simulink model "sampleModel228"  (R2021b)
settings: Solver=VariableStepAuto  StartTime=0.0  StopTime=10.0  RelTol=1e-3
undefined symbols (not defined in the file or in its folder): DiscIntNeverNeededParam
settings Model: Creator=user  LastModifiedBy=user

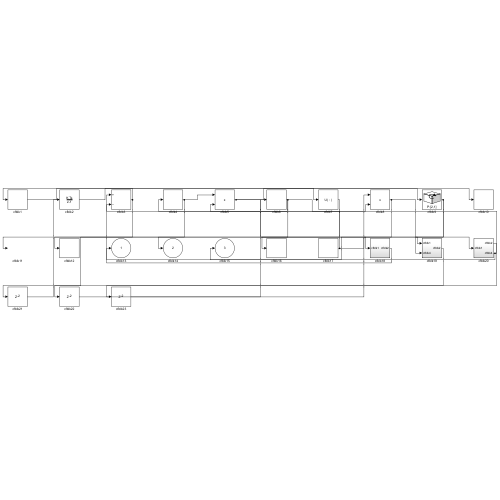
[thumbnail: Simulink's stored preview of the top-level diagram]
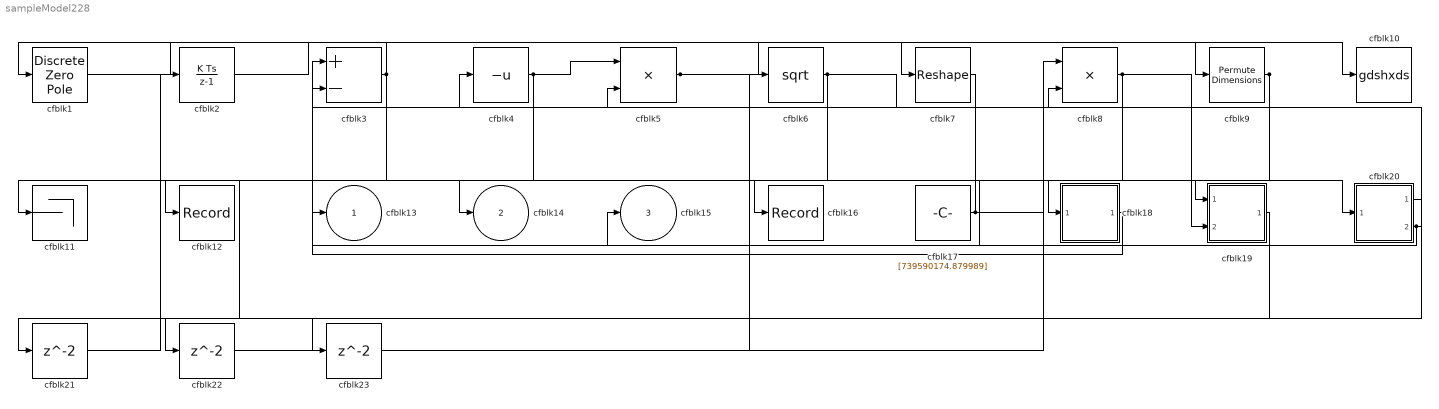
== system sampleModel228 ==
  cfblk1 : DiscreteZeroPole  Poles=[0 0.5]  Gain=1
  cfblk10 : ToWorkspace  VariableName=gdshxds  SaveFormat=Timeseries  SampleTime=-1
  cfblk11 : Terminator
  cfblk12 : Record  FileSettingsInternal="{\"entries\":[{\"content\":{\"excelSettings\":{\"content\":{},\"type\":\"Streamout.ExcelSettings\"}},\"type\":\"Streamout.FileSettingStorage\",\"uuid\":\"b7853067-aa81-4ff4-b03c-5eefb2e9456f\"}],\"packageUris\":[\"http://schema.mathworks.com/mf0/streamout_blocks/R2020a\"],\"version\":\"1.0\"}"  SignalsInternal="{\"entries\":[{\"content\":{\"signals\":[{\"content\":{\"blockPath\":[\"sampleModel228/cfblk12\"],\"channel\":[],\"dimensions\":[1,1],\"domain\":\"sampleModel228/cfblk12\",\"lineColor\":\"#edb120\",\"plots\":[1],\"port\":1,\"sid\":[\"\"],\"signalID\":8909,\"signalName\":\"cfblk3\"},\"type\":\"RecordBlkView.Signal\",\"uuid\":\"a36b1164-e6c3-447c-bebc-b7c5e35fa2b4\"}]},\"type\":\"RecordBlkView.InputSignals\",\"uuid\":\"7dc5b746-0d92-4986-ba98-2d25609e5927\"}],\"packageUris\":[\"http://schema.mathworks.com/mf0/streamout_blocks/R2020a\"],\"version\":\"1.0\"}"  VisualizationBindings="{\"sparklinesplugin\":{\"info\":[{\"bindingParametersList\":[],\"subplotID\":1}]}}"
  cfblk16 : Record  FileSettingsInternal="{\"entries\":[{\"content\":{\"excelSettings\":{\"content\":{},\"type\":\"Streamout.ExcelSettings\"}},\"type\":\"Streamout.FileSettingStorage\",\"uuid\":\"8bc86539-756b-41d3-8148-bbd2c8c8e0a7\"}],\"packageUris\":[\"http://schema.mathworks.com/mf0/streamout_blocks/R2020a\"],\"version\":\"1.0\"}"  SignalsInternal="{\"entries\":[{\"content\":{\"signals\":[{\"content\":{\"blockPath\":[\"sampleModel228/cfblk16\"],\"channel\":[],\"dimensions\":[1],\"domain\":\"sampleModel228/cfblk16\",\"lineColor\":\"#7e2f8e\",\"plots\":[1],\"port\":1,\"sid\":[\"\"],\"signalID\":8913,\"signalName\":\"cfblk6\"},\"type\":\"RecordBlkView.Signal\",\"uuid\":\"a333abe5-6e46-4828-b4fc-efe21365cda2\"}]},\"type\":\"RecordBlkView.InputSignals\",\"uuid\":\"23a0d02e-941f-4979-b7cc-281993342506\"}],\"packageUris\":[\"http://schema.mathworks.com/mf0/streamout_blocks/R2020a\"],\"version\":\"1.0\"}"  VisualizationBindings="{\"sparklinesplugin\":{\"info\":[{\"bindingParametersList\":[],\"subplotID\":1}]}}"
  cfblk17 : Constant  Value=[739590174.879989]  SampleTime=1
  cfblk18 : Subsystem
  cfblk19 : Subsystem
  cfblk2 : DiscreteIntegrator  ICPrevOutput=DiscIntNeverNeededParam  ICPrevScaledInput=DiscIntNeverNeededParam
  cfblk20 : Subsystem
  cfblk21 : Delay  SampleTime=1
  cfblk22 : Delay  SampleTime=1
  cfblk23 : Delay  SampleTime=1
  cfblk3 : Sum  Inputs=+-
  cfblk4 : UnaryMinus
  cfblk5 : Product
  cfblk6 : Sqrt  SaturateOnIntegerOverflow=on
  cfblk7 : Reshape
  cfblk8 : Product  Inputs=**
  cfblk9 : PermuteDimensions
  cfblk13 : Outport
  cfblk14 : Outport  Port=2
  cfblk15 : Outport  Port=3
  wires:
  cfblk1/1 -> cfblk7/1
  cfblk7/1 -> cfblk14/1
  cfblk9/1 -> cfblk15/1, cfblk19/2(cfblk4)
  cfblk17/1 -> cfblk4/1, cfblk19/1(cfblk1)
  cfblk18/1(cfblk2) -> cfblk3/1
  cfblk5/1 -> cfblk10/1, cfblk18/1(cfblk1)
  cfblk4/1 -> cfblk5/1, cfblk11/1
  cfblk3/1 -> cfblk12/1, cfblk1/1
  cfblk20/2(cfblk4) -> cfblk3/2, cfblk13/1
  cfblk8/1 -> cfblk20/1(cfblk1), cfblk22/1
  cfblk6/1 -> cfblk5/2, cfblk16/1, cfblk8/2
  cfblk2/1 -> cfblk9/1
  cfblk19/1(cfblk2) -> cfblk21/1
  cfblk21/1 -> cfblk2/1
  cfblk22/1 -> cfblk6/1
  cfblk20/1(cfblk2) -> cfblk23/1
  cfblk23/1 -> cfblk8/1

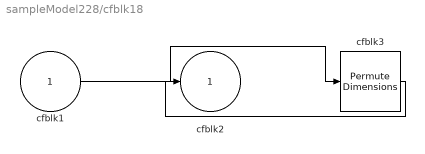
== system sampleModel228/cfblk18 ==
  cfblk1 : Inport
  cfblk3 : PermuteDimensions
  cfblk2 : Outport
  wires:
  cfblk1/1 -> cfblk3/1
  cfblk3/1 -> cfblk2/1

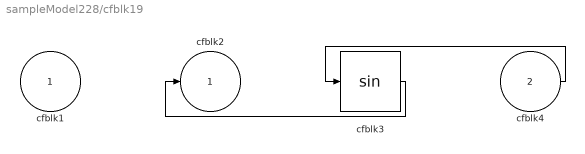
== system sampleModel228/cfblk19 ==
  cfblk1 : Inport
  cfblk4 : Inport  Port=2
  cfblk3 : Trigonometry
  cfblk2 : Outport
  wires:
  cfblk4/1 -> cfblk3/1
  cfblk3/1 -> cfblk2/1

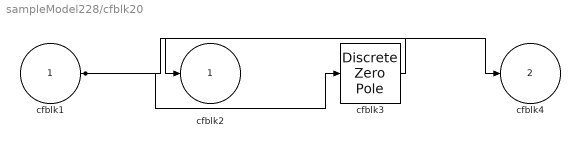
== system sampleModel228/cfblk20 ==
  cfblk1 : Inport
  cfblk3 : DiscreteZeroPole  Poles=[0 0.5]  Gain=1
  cfblk2 : Outport
  cfblk4 : Outport  Port=2
  wires:
  cfblk3/1 -> cfblk2/1
  cfblk1/1 -> cfblk3/1, cfblk4/1
